simulink model "ooknrzbw"  (Simulink 5.0)
settings: Solver=ode45  StartTime=0.0  StopTime=999999  MaxStep=0.05  MinStep=.000001  RelTol=1e-3  AbsTol=1e-3
undefined symbols (not defined in the file or in its folder): eyediasi, eyesampl, sbiterr
libraries: librnew x2
CloseFcn:
  | closemodcross
settings Model: Creator=gerhard  LastModifiedBy=bauch  ExtModeAutoUpdateStatusClock=off  SaveTime=off  SaveOutput=off  BlockReductionOpt=off  BooleanDataType=off

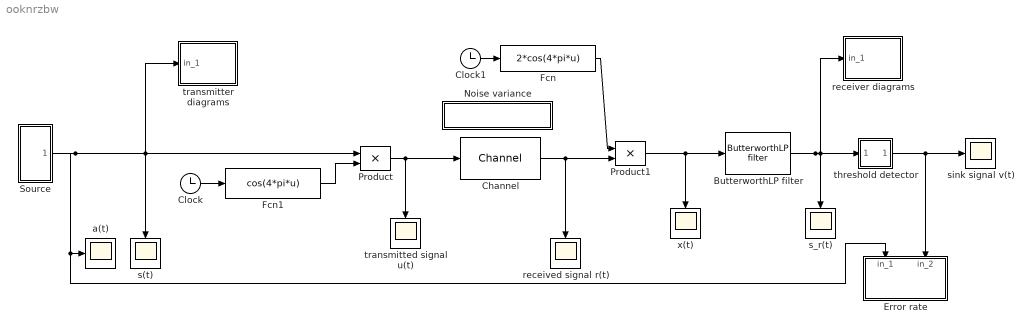
== system ooknrzbw ==
  ButterworthLP filter : librnew/ButterworthLP filter  n=4  MaskParam1=5
  Channel : librnew/Channel  m=0  variance=0.001  s=12345
  Clock : Clock
      settings: Decimation=10
  Clock1 : Clock
      settings: Decimation=10
  Error rate : Subsystem  Orientation=down  LoadFcn=sbiterr([],[],[],'LoadBlock')  StartFcn=sbiterr([],[],[],'Start')  StopFcn=sbiterr([],[],[],'Stop')  mask(Symbol/bit error counter){@1=1, @2=10, @3=1, @4=1}
      mask prompts: @1 "Bit per symbol:"; @2 "Number of digits on display:"; @3 "Delay between 1st port and 2nd port:"; @4 "Sample time (sec):"
      mask help: Use the input data from the 1st port as the reference signal to detect the number of errors and error rate of the 2nd signal.
      mask init:
      | K=@1;num_lin=@2;TDelay=@3;Sample=@4;
      settings: CopyFcn=sbiterr([],[],[],'CopyBlock')  DeleteFcn=sbiterr([],[],[],'DeleteBlock')  NameChangeFcn=sbiterr([],[],[],'NameChange')
      mask Help: The signal from the first port must be a scalar. The second input port can be a vector with a delay to the first port signal. The comparison happens only at the sampling point.
      mask Display: disp('Error\nmeter')
  Fcn : Fcn  Expr=2*cos(4*pi*u)
  Fcn1 : Fcn  Expr=cos(4*pi*u)
  Noise variance : Subsystem
      settings: OpenFcn=setnoise
      mask Type: noise
      mask Display: disp('Noise variance')
  Product : Product  SaturateOnIntegerOverflow=on  InputSameDT=on
  Product1 : Product  SaturateOnIntegerOverflow=on  InputSameDT=on
  Source : Subsystem
  a(t) : Scope
      settings: TimeRange=25.000000  YMin=-2  YMax=2  DataFormat=Array
  received signal r(t) : Scope
      settings: Orientation=down  TimeRange=25.000000  YMin=-2  YMax=2  DataFormat=Array
  receiver diagrams : Subsystem  mask(Diagrams){starttime=1, anzahl=40, offset=.075}
      mask prompts: starttime "Plot start time:"; anzahl "Samples per time slot (2*T):"; offset "Decision offset:"
      mask help: Eye pattern, signal space trajectory and scatter plot
      mask init:
      | [x, y] = srcsicon(10);
      mask Display: plot(0,0,100,100,x,y)
  s(t) : Scope
      settings: Orientation=down  TimeRange=25.000000  YMin=-2  YMax=2  DataFormat=Array
  s_r(t) : Scope
      settings: Orientation=down  TimeRange=25.000000  YMin=-2  YMax=2  DataFormat=Array
  sink signal v(t) : Scope
      settings: TimeRange=25.000000  YMin=-2  YMax=2  DataFormat=Array
  threshold detector : Subsystem
      mask Type: Sign
      mask Description: y = sign(x)
      mask Help: Sign Function:\n\t\t\ty = 1 if x > 0\n\t\t\ty = 0 if x = 0\n\t\t\ty = -1 if x < 0
      mask Display: plot(-50,-50,50,50,[-50,50],[0,0],[0,0],[-50,50],[-40,0],[-30,-30],[0,40],[30,30])
  transmitted signal u(t) : Scope
      settings: Orientation=down  TimeRange=25.000000  YMin=-2  YMax=2  DataFormat=Array
  transmitter diagrams : Subsystem  mask(Diagrams){starttime=0, anzahl=40, offset=0}
      mask prompts: starttime "Plot start time:"; anzahl "Samples per time slot (2*T):"; offset "Decision offset:"
      mask help: Eye pattern, signal space trajectory and scatter plot.
      mask init:
      | [x, y] = srcsicon(10);
      mask Display: plot(0,0,100,100,x,y)
  x(t) : Scope
      settings: Orientation=down  TimeRange=25.000000  YMin=-2  YMax=2  DataFormat=Array
  wires:
  Clock/1 -> Fcn1/1
  Fcn/1 -> Product1/1
  Clock1/1 -> Fcn/1
  Product1/1 -> x(t)/1, ButterworthLP filter/1
  ButterworthLP filter/1 -> s_r(t)/1, receiver diagrams/1(in_1), threshold detector/1(in_1)
  threshold detector/1(out_1) -> sink signal v(t)/1, Error rate/2(in_2)
  Fcn1/1 -> Product/2
  Product/1 -> transmitted signal u(t)/1, Channel/1
  Channel/1 -> Product1/2, received signal r(t)/1
  Source/1(out_1) -> Product/1, transmitter diagrams/1(in_1), s(t)/1, a(t)/1, Error rate/1(in_1)

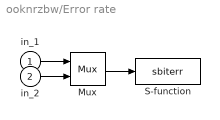
== system ooknrzbw/Error rate ==
  in_1 : Inport
  in_2 : Inport  Port=2
  Mux : Mux  Inputs=2
  S-function : S-Function  FunctionName=sbiterr  Parameters=num_lin, K, TDelay, Sample
  wires:
  in_2/1 -> Mux/2
  in_1/1 -> Mux/1
  Mux/1 -> S-function/1

== system ooknrzbw/Noise variance ==

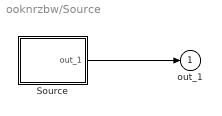
== system ooknrzbw/Source ==
  Source : Subsystem  mask(Read from workspace){@1=randint(1000,1,2), @2=1, @3=1, @4=1}
      mask prompts: @1 "Variable (column_number=block_output_length):"; @2 "Data output sample time (sec):"; @3 "Repeat flag (1: repeat read, 0: output zeros after eof)."; @4 "Initial output:"
      mask help:
      | Read from a workspace variable at
      | sampling time point.
      mask init:
      | var=@1;td=@2;ts=td(1);if (length(td)>=2),off=td(2);else off=0;end;cyc=@3;ini=@4;[x,y]=srcsicon(7);
      mask Help: This block reads from a workspace variable at a given sample time. The column number is the block output vector length. When the simulation reaches the end of the variable (eof), the block will cyclically output from the first row of the variable or output zeros based on the repeat flag entree.
      mask Display: plot(0,0,100,100,x,y);disp('Rd wksp')
  out_1 : Outport
  wires:
  Source/1(out_1) -> out_1/1

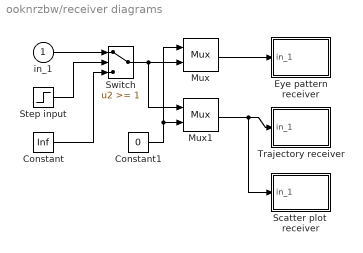
== system ooknrzbw/receiver diagrams ==
  in_1 : Inport
  Constant : Constant  Value=Inf
  Constant1 : Constant  Value=0
  Eye pattern receiver : Subsystem  LoadFcn=eyesampl([],[],[],'LoadBlock')  StartFcn=eyesampl([],[],[],'Start')  StopFcn=eyesampl([],[],[],'Stop')  mask(Eye-diagram/scatter plot){@1=[2 0 1+offset], @2=[-1.5 1.5], @3=0, @4='w-/r-', @5=0, @6=2/anzahl}
      mask prompts: @1 "[Symbol interval, plot offset, decision point offset]:"; @2 "Lower and upper bound of in-coming signal (1x2 vector):"; @3 "Number of saved traces:"; @4 "Line-type for eye-pattern diagram (0 for no plot):"; @5 "Line-type for scatter plot (0 for no plot):"; @6 "Plot update sample time:"
      mask help: Produce eye-pattern diagram and/or scatter plot.
      mask init:
      | time_range=@1;boundary=@2;kept_length=@3;eye_line=@4;scatter_line=@5;two_d_line=@6;[x,y]=srcsicon(10);
      settings: CopyFcn=eyesampl([],[],[],'CopyBlock')  DeleteFcn=eyesampl([],[],[],'DeleteBlock')  NameChangeFcn=eyesampl([],[],[],'NameChange')
      mask Help: This plot opens one, or two plots by assigning the line type parameters. The scatter plot point is selected by the decision point in the first parameter entry. A decision line is drawn in the eye-pattern diagram. The plot is updated at the plot update sample time point.
      mask Display: plot(0,0,100,100,x,y);
  Mux : Mux  Inputs=2
  Mux1 : Mux  Inputs=2
  Scatter plot  receiver : Subsystem  LoadFcn=eyesampl([],[],[],'LoadBlock')  StartFcn=eyesampl([],[],[],'Start')  StopFcn=eyesampl([],[],[],'Stop')  mask(Eye-diagram/scatter plot){@1=[1 .5 .999], @2=[-1.5 1.5], @3=0, @4=0, @5='b.', @6=[.5 offset]}
      mask prompts: @1 "[Symbol interval, plot offset, decision point offset]:"; @2 "Lower and upper bound of in-coming signal (1x2 vector):"; @3 "Number of saved traces:"; @4 "Line-type for eye-pattern diagram (0 for no plot):"; @5 "Line-type for scatter plot (0 for no plot):"; @6 "Plot update sample time:"
      mask help: Produce eye-pattern diagram and/or scatter plot.
      mask init:
      | time_range=@1;boundary=@2;kept_length=@3;eye_line=@4;scatter_line=@5;two_d_line=@6;[x,y]=srcsicon(10);
      settings: CopyFcn=eyesampl([],[],[],'CopyBlock')  DeleteFcn=eyesampl([],[],[],'DeleteBlock')  NameChangeFcn=eyesampl([],[],[],'NameChange')
      mask Help: This plot opens one, or two plots by assigning the line type parameters. The scatter plot point is selected by the decision point in the first parameter entry. A decision line is drawn in the eye-pattern diagram. The plot is updated at the plot update sample time point.
      mask Display: plot(0,0,100,100,x,y);
  Step input : Step  Time=starttime  SampleTime=1
  Switch : Switch  Threshold=1  SaturateOnIntegerOverflow=on  InputSameDT=on
  Trajectory receiver : Subsystem  LoadFcn=eyediasi([],[],[],'LoadBlock')  StartFcn=eyediasi([],[],[],'Start')  StopFcn=eyediasi([],[],[],'Stop')  mask(Eye-diagram/scatter plot){@1=[2 0 1], @2=[-1.5 1.5], @3=0, @4=0, @5=0, @6='g-'}
      mask prompts: @1 "Eye-pattern plot time frame:"; @2 "Lower and upper bound of in-coming signal (1x2 vector):"; @3 "Number of saved traces:"; @4 "Line-type for eye-pattern diagram (0 for no plot):"; @5 "Line-type for scatter plot (0 for no plot):"; @6 "Line-type for x-y plot (0 for no plot):"
      mask help:
      | Produce eye-pattern diagram/scatter
      | plot/x-y plot with the rising edge of the second input as the decision line.
      mask init:
      | time_range=@1;boundary=@2;kept_length=@3;eye_line=@4;scatter_line=@5;two_d_line=@6;[x,y]=srcsicon(10);[v,w]=trigicon(0,25,get_param(gcb,'orientation'),2);
      settings: CopyFcn=eyediasi([],[],[],'CopyBlock')  DeleteFcn=eyediasi([],[],[],'DeleteBlock')  NameChangeFcn=eyediasi([],[],[],'NameChange')
      mask Help: This plot opens one, two, or three plots by assigning the line type parameters. The scatter plot point is selected by the rising edge of a trigger signal. A decision line is drawn at the rising edge of the trigger signal.
      mask Display: plot(0,0,100,100,x,y,v,w);
  wires:
  Mux/1 -> Eye pattern receiver/1(in_1)
  in_1/1 -> Switch/1
  Step input/1 -> Switch/2
  Constant/1 -> Switch/3
  Mux1/1 -> Trajectory receiver/1(in_1), Scatter plot  receiver/1(in_1)
  Constant1/1 -> Mux/1, Mux1/2
  Switch/1 -> Mux/2, Mux1/1

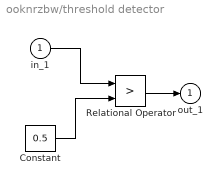
== system ooknrzbw/threshold detector ==
  in_1 : Inport
  Constant : Constant  Value=0.5
  Relational Operator : RelationalOperator  Operator=>  InputSameDT=on
  out_1 : Outport
  wires:
  Relational Operator/1 -> out_1/1
  Constant/1 -> Relational Operator/2
  in_1/1 -> Relational Operator/1

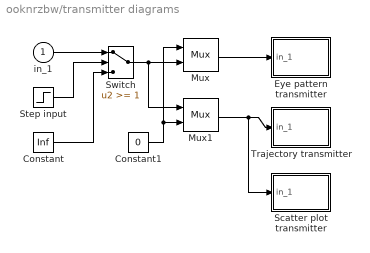
== system ooknrzbw/transmitter diagrams ==
  in_1 : Inport
  Constant : Constant  Value=Inf
  Constant1 : Constant  Value=0
  Eye pattern transmitter : Subsystem  LoadFcn=eyesampl([],[],[],'LoadBlock')  StartFcn=eyesampl([],[],[],'Start')  StopFcn=eyesampl([],[],[],'Stop')  mask(Eye-diagram/scatter plot){@1=[2 0 1+offset], @2=[-1.5 1.5], @3=0, @4='w-/r-', @5=0, @6=2/anzahl}
      mask prompts: @1 "[Symbol interval, plot offset, decision point offset]:"; @2 "Lower and upper bound of in-coming signal (1x2 vector):"; @3 "Number of saved traces:"; @4 "Line-type for eye-pattern diagram (0 for no plot):"; @5 "Line-type for scatter plot (0 for no plot):"; @6 "Plot update sample time:"
      mask help: Produce eye-pattern diagram and/or scatter plot.
      mask init:
      | time_range=@1;boundary=@2;kept_length=@3;eye_line=@4;scatter_line=@5;two_d_line=@6;[x,y]=srcsicon(10);
      settings: CopyFcn=eyesampl([],[],[],'CopyBlock')  DeleteFcn=eyesampl([],[],[],'DeleteBlock')  NameChangeFcn=eyesampl([],[],[],'NameChange')
      mask Help: This plot opens one, or two plots by assigning the line type parameters. The scatter plot point is selected by the decision point in the first parameter entry. A decision line is drawn in the eye-pattern diagram. The plot is updated at the plot update sample time point.
      mask Display: plot(0,0,100,100,x,y);
  Mux : Mux  Inputs=2
  Mux1 : Mux  Inputs=2
  Scatter plot transmitter : Subsystem  LoadFcn=eyesampl([],[],[],'LoadBlock')  StartFcn=eyesampl([],[],[],'Start')  StopFcn=eyesampl([],[],[],'Stop')  mask(Eye-diagram/scatter plot){@1=[1 .5 .999], @2=[-1.5 1.5], @3=0, @4=0, @5='b.', @6=[.5 offset]}
      mask prompts: @1 "[Symbol interval, plot offset, decision point offset]:"; @2 "Lower and upper bound of in-coming signal (1x2 vector):"; @3 "Number of saved traces:"; @4 "Line-type for eye-pattern diagram (0 for no plot):"; @5 "Line-type for scatter plot (0 for no plot):"; @6 "Plot update sample time:"
      mask help: Produce eye-pattern diagram and/or scatter plot.
      mask init:
      | time_range=@1;boundary=@2;kept_length=@3;eye_line=@4;scatter_line=@5;two_d_line=@6;[x,y]=srcsicon(10);
      settings: CopyFcn=eyesampl([],[],[],'CopyBlock')  DeleteFcn=eyesampl([],[],[],'DeleteBlock')  NameChangeFcn=eyesampl([],[],[],'NameChange')
      mask Help: This plot opens one, or two plots by assigning the line type parameters. The scatter plot point is selected by the decision point in the first parameter entry. A decision line is drawn in the eye-pattern diagram. The plot is updated at the plot update sample time point.
      mask Display: plot(0,0,100,100,x,y);
  Step input : Step  Time=starttime  SampleTime=1
  Switch : Switch  Threshold=1  SaturateOnIntegerOverflow=on  InputSameDT=on
  Trajectory transmitter : Subsystem  LoadFcn=eyediasi([],[],[],'LoadBlock')  StartFcn=eyediasi([],[],[],'Start')  StopFcn=eyediasi([],[],[],'Stop')  mask(Eye-diagram/scatter plot){@1=[2 0 1], @2=[-1.5 1.5], @3=0, @4=0, @5=0, @6='g-'}
      mask prompts: @1 "Eye-pattern plot time frame:"; @2 "Lower and upper bound of in-coming signal (1x2 vector):"; @3 "Number of saved traces:"; @4 "Line-type for eye-pattern diagram (0 for no plot):"; @5 "Line-type for scatter plot (0 for no plot):"; @6 "Line-type for x-y plot (0 for no plot):"
      mask help:
      | Produce eye-pattern diagram/scatter
      | plot/x-y plot with the rising edge of the second input as the decision line.
      mask init:
      | time_range=@1;boundary=@2;kept_length=@3;eye_line=@4;scatter_line=@5;two_d_line=@6;[x,y]=srcsicon(10);[v,w]=trigicon(0,25,get_param(gcb,'orientation'),2);
      settings: CopyFcn=eyediasi([],[],[],'CopyBlock')  DeleteFcn=eyediasi([],[],[],'DeleteBlock')  NameChangeFcn=eyediasi([],[],[],'NameChange')
      mask Help: This plot opens one, two, or three plots by assigning the line type parameters. The scatter plot point is selected by the rising edge of a trigger signal. A decision line is drawn at the rising edge of the trigger signal.
      mask Display: plot(0,0,100,100,x,y,v,w);
  wires:
  Switch/1 -> Mux/2, Mux1/1
  Constant1/1 -> Mux/1, Mux1/2
  Mux1/1 -> Trajectory transmitter/1(in_1), Scatter plot transmitter/1(in_1)
  Constant/1 -> Switch/3
  Step input/1 -> Switch/2
  in_1/1 -> Switch/1
  Mux/1 -> Eye pattern transmitter/1(in_1)

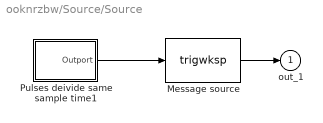
== system ooknrzbw/Source/Source ==
  Message source : S-Function  FunctionName=trigwksp  Parameters=var,thd,cyclFlag,ini  mask(Read from workspace){@1=var, @2=.1, @3=cyc, @4=ini}
      mask prompts: @1 "Read the variable:"; @2 "Threshold for the input pulse:"; @3 "Cyclic read variable (1) or amend zeros (0)."; @4 "Output before first trigger:"
      mask help: The raising edge of input pulse trigger the block output the next row from the workspace variable.
      mask init:
      | var=@1;thd=@2;cyclFlag=@3;ini=@4;
      mask Help: This block reads the data from a workspace variable. The output is refreshed at the raising edge of the input pulse.
      mask Display: disp('Triggered\nread')
  Pulses deivide same sample time1 : Subsystem  mask(Pulse generator){@1=ts, @2=1, @3=off}
      mask prompts: @1 "Sample time (scalar, sec):"; @2 "Divider (integer vector):"; @3 "Offset (have same dimension as Divider:"
      mask help: Vector pulses with sample rate of each pulse as Sample_time ./Divider.
      mask init:
      | samp_time=@1;out_divid=@2;offset=@3;
      mask Help: This block generator a vector pulses. The output length is the same as the vector defined in "Divider". The ith element of the output has the sample time Sample_time/Divider(i). All elements in "Divider" must be integers.
      mask Display: disp('Vector\nPulse')
  out_1 : Outport
  wires:
  Message source/1 -> out_1/1
  Pulses deivide same sample time1/1(Outport) -> Message source/1

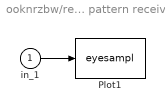
== system ooknrzbw/receiver diagrams/Eye pattern receiver ==
  in_1 : Inport
  Plot1 : S-Function  FunctionName=eyesampl  Parameters=time_range, boundary, kept_length, eye_line, scatter_line, two_d_line
  wires:
  in_1/1 -> Plot1/1

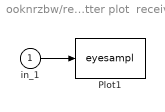
== system ooknrzbw/receiver diagrams/Scatter plot  receiver ==
  in_1 : Inport
  Plot1 : S-Function  FunctionName=eyesampl  Parameters=time_range, boundary, kept_length, eye_line, scatter_line, two_d_line
  wires:
  in_1/1 -> Plot1/1

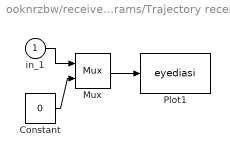
== system ooknrzbw/receiver diagrams/Trajectory receiver ==
  in_1 : Inport
  Constant : Constant  Value=0
  Mux : Mux  Inputs=2
  Plot1 : S-Function  FunctionName=eyediasi  Parameters=time_range, boundary, kept_length, eye_line, scatter_line, two_d_line
  wires:
  Mux/1 -> Plot1/1
  Constant/1 -> Mux/2
  in_1/1 -> Mux/1

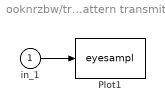
== system ooknrzbw/transmitter diagrams/Eye pattern transmitter ==
  in_1 : Inport
  Plot1 : S-Function  FunctionName=eyesampl  Parameters=time_range, boundary, kept_length, eye_line, scatter_line, two_d_line
  wires:
  in_1/1 -> Plot1/1

== system ooknrzbw/transmitter diagrams/Scatter plot transmitter ==
  in_1 : Inport
  Plot1 : S-Function  FunctionName=eyesampl  Parameters=time_range, boundary, kept_length, eye_line, scatter_line, two_d_line
  wires:
  in_1/1 -> Plot1/1

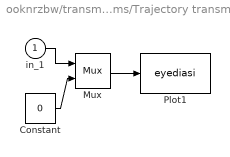
== system ooknrzbw/transmitter diagrams/Trajectory transmitter ==
  in_1 : Inport
  Constant : Constant  Value=0
  Mux : Mux  Inputs=2
  Plot1 : S-Function  FunctionName=eyediasi  Parameters=time_range, boundary, kept_length, eye_line, scatter_line, two_d_line
  wires:
  in_1/1 -> Mux/1
  Constant/1 -> Mux/2
  Mux/1 -> Plot1/1

== system ooknrzbw/Source/Source/Pulses deivide same sample time1 ==
  S-function1 : S-Function  FunctionName=homopuls  Parameters=samp_time, out_divid, offset
  Outport : Outport
  wires:
  S-function1/1 -> Outport/1
